simulink model "CFBTTCQIED"  (R2021b)
settings: Solver=ode23t  StartTime=0.0  StopTime=simtime  RelTol=1e-3
values from neighbouring files (symbols this model uses):
  a1 = (Iyy-Izz)/Ixx    (= -0.733333333333)    [CFBTTCQIED.m]
  a1_p = 1    [CFBTTCQIED.m]
  a1_r = 1    [CFBTTCQIED.m]
  a1_x = 1    [CFBTTCQIED.m]
  a1_y = 1    [CFBTTCQIED.m]
  a1_z = 1    [CFBTTCQIED.m]
  a2 = Jr/Ixx    (= 0.008)    [CFBTTCQIED.m]
  a2_r = 2    [CFBTTCQIED.m]
  a2_x = 2    [CFBTTCQIED.m]
  a2_y = 2    [CFBTTCQIED.m]
  a2_z = 2    [CFBTTCQIED.m]
  a3 = (Izz-Ixx)/Iyy    (= 0.733333333333)    [CFBTTCQIED.m]
  a4 = Jr/Iyy    (= 0.008)    [CFBTTCQIED.m]
  a5 = (Ixx-Iyy)/Izz    (= 0)    [CFBTTCQIED.m]
  b = 3.13e-5    (= 3.13e-05)    [CFBTTCQIED.m]
  b1 = l/Ixx    (= 30.6666666667)    [CFBTTCQIED.m]
  b2 = l/Iyy    (= 30.6666666667)    [CFBTTCQIED.m]
  b3 = l/Izz    (= 17.6923076923)    [CFBTTCQIED.m]
  d = 7.5e-7    (= 7.5e-07)    [CFBTTCQIED.m]
  epsi = 0.00001    (= 1e-05)    [CFBTTCQIED.m]
  g = 9.81    [CFBTTCQIED.m]
  init_cond_pitch = 0    [CFBTTCQIED.m]
  init_cond_roll = 0    [CFBTTCQIED.m]
  init_cond_x = 0    [CFBTTCQIED.m]
  init_cond_y = 2    [CFBTTCQIED.m]
  init_cond_yaw = 0    [CFBTTCQIED.m]
  init_cond_z = 0    [CFBTTCQIED.m]
  k = 2.980e-6    (= 2.98e-06)    [CFBTTCQIED.m]
  lambda = zxc    (= 10)    [CFBTTCQIED.m]
  lambda_x = 2    [CFBTTCQIED.m]
  lambda_y = 2    [CFBTTCQIED.m]
  lambda_z = 2    [CFBTTCQIED.m]
  lamda_phi = zxc    (= 10)    [CFBTTCQIED.m]
  lamda_psi = zxc    (= 10)    [CFBTTCQIED.m]
  lamda_theta = zxc    (= 10)    [CFBTTCQIED.m]
  m = 0.650    (= 0.65)    [CFBTTCQIED.m]
  Omega_r = 1    [CFBTTCQIED.m]
  p1_phi = 20    [CFBTTCQIED.m]
  p1_psi = 20    [CFBTTCQIED.m]
  p1_theta = 20    [CFBTTCQIED.m]
  p1_x = 2    [CFBTTCQIED.m]
  p1_y = 2    [CFBTTCQIED.m]
  p1_z = 2    [CFBTTCQIED.m]
  p2_phi = 5    [CFBTTCQIED.m]
  p2_psi = 5    [CFBTTCQIED.m]
  p2_theta = 5    [CFBTTCQIED.m]
  p2_x = 2    [CFBTTCQIED.m]
  p2_y = 2    [CFBTTCQIED.m]
  p2_z = 2    [CFBTTCQIED.m]
  psi_des = yaw_des    (= 0.523598775598)    [CFBTTCQIED.m]
  sample_time_pitch = 15    [CFBTTCQIED.m]
  sample_time_roll = 15    [CFBTTCQIED.m]
  sample_time_yaw = 1    [CFBTTCQIED.m]
  tau = 0.1    [CFBTTCQIED.m]
libraries: simulink x2
(part 2 of 2)

== matlab function CFBTTCQIED/MATLAB Function ==
  data: d_phi input; d_theta input; d_psi input; phi_des input; theta_des input; psi_des input; phi_des_dot input; theta_des_dot input; psi_des_dot input; phi input; U2 output; theta input; psi input; phi_dot input; theta_dot input; psi_dot input; p1_phi input; p1_theta input; p1_psi input; p2_phi input; p2_theta input; p2_psi input; U3 output; U4 output; xi_phi input; xi_theta input; xi_psi input; mu_phi output; mu_theta output; mu_psi output
function [U2,U3,U4,mu_phi,mu_theta,mu_psi] = fcn(d_phi,d_theta,d_psi,phi_des,theta_des,psi_des,phi_des_dot,theta_des_dot,psi_des_dot,phi,theta,psi,phi_dot,theta_dot,psi_dot,p1_phi,p1_theta,p1_psi,p2_phi,p2_theta,p2_psi,xi_phi,xi_theta,xi_psi)
%%
g = 9.81;                % Gravity                    [m/sec^2]     
m = 0.650;               % Mass                       [kg]     
l = 0.23;                % Length                     [m]
k = 2.980e-6;            %
b = 3.13e-5;             % Thrust coefficient         [N.sec^2]
d = 7.5e-7;              % Drag coefficient           [Nm.sec^2]
R_rad = 0.15;            % Properller radius          [m]
c = 0.04;                % Properller chord           [m]
Jr = 6e-5;               % Rotor inertia              [kg.m^2]

Im = 3.357e-5;           %
Ixx = 7.5e-3;            % Inertia on x-axis          [kg.m^2]
Iyy = 7.5e-3;            % Inertia on y-axis          [kg.m^2]
Izz = 1.3e-2;            % Inertia on z-axis          [kg.m^2]

Omega_r = 1;             % Residual angular speed of propeller     [rad.sec]
% Parameters simplification
a1 = (Iyy-Izz)/Ixx;
a2 = Jr/Ixx;
b1 = l/Ixx;


a3 = (Izz-Ixx)/Iyy;
a4 = Jr/Iyy;
b2 = l/Iyy;

a5 = (Ixx-Iyy)/Izz;
b3 = l/Izz;
%%
% z1
z1 =     phi - phi_des ;
z3 =    theta - theta_des  ;
z5 =     psi - psi_des ;

% z2
z2 = phi_dot - phi_des_dot - xi_phi;
z4 = theta_dot - theta_des_dot - xi_theta;
z6 = psi_dot - psi_des_dot - xi_psi;

% mu
mu_phi =  - p1_phi*z1 + phi_des_dot;
mu_theta =  - p1_theta*z3 + theta_des_dot;
mu_psi =  - p1_psi*z5 + psi_des_dot;

% control inputs
U2 = -(a1*theta_dot*psi_dot + a2*Omega_r*theta_dot -  xi_phi + p2_phi*z2 + z1 + d_phi)/b1;
U3 = -(a3*phi_dot*psi_dot - a4*Omega_r*phi_dot - xi_theta+ p2_theta*z4 + z3 + d_theta)/b2;
U4 = -(a5*theta_dot*phi_dot    - xi_psi + p2_psi*z6 + z5 + d_psi)/b3;
y = [U2,U3,U4,mu_phi,mu_theta,mu_psi];

== matlab function CFBTTCQIED/Subsystem2/MATLAB Function2 ==
  data: dx input; dy input; dz input; Ux output; x input; y input; z input; x_dot input; y_dot input; z_dot input; x_des input; y_des input; z_des input; x_des_dot input; y_des_dot input; z_des_dot input; p1_x input; p1_y input; p1_z input; p2_x input; p2_y input; p2_z input; Uy output; Uz output; xi_x input; xi_y input; xi_z input; mu_x output; mu_y output; mu_z output
function [Ux,Uy,Uz,mu_x,mu_y,mu_z] = fcn(dx,dy,dz,x,y,z,x_dot,y_dot,z_dot,x_des,y_des,z_des,x_des_dot,y_des_dot,z_des_dot,p1_x,p1_y,p1_z,p2_x,p2_y,p2_z,xi_x,xi_y,xi_z)
% Parameters
g = 9.81;                % Gravity                    [m/sec^2]     
m = 0.650;               % Mass                       [kg]     
l = 0.23;                % Length                     [m]
k = 2.980e-6;            %
b = 3.13e-5;             % Thrust coefficient         [N.sec^2]
d = 7.5e-7;              % Drag coefficient           [Nm.sec^2]
R_rad = 0.15;            % Properller radius          [m]
c = 0.04;                % Properller chord           [m]
Jr = 6e-5;               % Rotor inertia              [kg.m^2]

Im = 3.357e-5;           %
Ixx = 7.5e-3;            % Inertia on x-axis          [kg.m^2]
Iyy = 7.5e-3;            % Inertia on y-axis          [kg.m^2]
Izz = 1.3e-2;            % Inertia on z-axis          [kg.m^2]

Omega_r = 1;             % Residual angular speed of propeller     [rad.sec]
% Parameters simplification
a1 = (Iyy-Izz)/Ixx;
a2 = Jr/Ixx;
b1 = l/Ixx;


a3 = (Izz-Ixx)/Iyy;
a4 = Jr/Iyy;
b2 = l/Iyy;

a5 = (Ixx-Iyy)/Izz;
b3 = l/Izz;
%% controllers
% z1
z1_x =   x- x_des  ;
z1_y =   y - y_des ;
z1_z =   z - z_des ;

% z2
z2_x = x_dot - x_des_dot - xi_x;
z2_y = y_dot - y_des_dot - xi_y;
z2_z = z_dot - z_des_dot - xi_z;


% mu
mu_x =  - p1_x*z1_x + x_des_dot;
mu_y =  - p1_y*z1_y + y_des_dot;
mu_z =  - p1_z*z1_z + z_des_dot;

% controllers

Ux = -( -  xi_x + p2_x*z2_x + z1_x+ dx );
Uy = -( - xi_y+ p2_y*z2_y + z1_y + dy );
Uz = -(   - xi_z + p2_z*z2_z + z1_z +dz);
y = [Ux,Uy,Uz,mu_x,mu_y,mu_z];
